simulink model "ballbeam_sim"  (Simulink 7.9)
settings: Solver=ode45  StartTime=0.0  StopTime=100  RelTol=1e-3
values from neighbouring files (symbols this model uses):
  kd_th = 2*zeta_th*wn_th/a1    [param.m]
  kd_z = -14*zeta_z*wn_z/(5*AP.g)    [param.m]
  kp_th = (AP.Fmax-Fe)/A_th    [param.m]
  kp_z = -A_th/A_z    [param.m]
undefined symbols (not defined in the file or in its folder): AP, drawBallBeam
settings Model: Creator=beard  LastModifiedBy=timmclain
settings OptimizationCC: InitFltsAndDblsToZero=on
settings DebuggingCC: FcnCallInpInsideContextMsg=Use local settings  StrictBusMsg=Warning
settings GRTTargetCC: CombineOutputUpdateFcns=off  GRTInterface=on

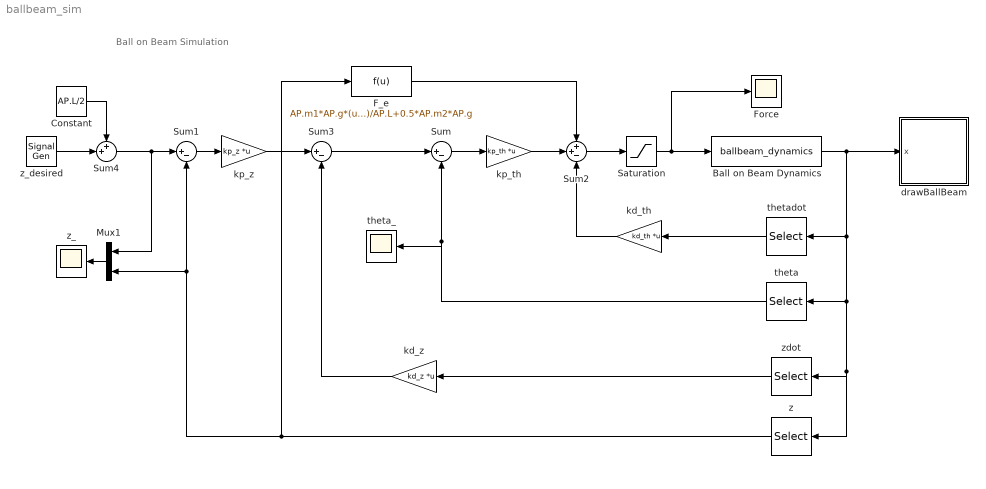
== system ballbeam_sim ==
  note: Ball on Beam Simulation
  Ball on Beam Dynamics : S-Function  FunctionName=ballbeam_dynamics  Parameters=AP  EnableBusSupport=off
  Constant : Constant  Value=AP.L/2
  F_e : Fcn  Expr=AP.m1*AP.g*(u)/AP.L+0.5*AP.m2*AP.g
  Force : Scope
      settings: TimeRange=100  YMin=6  YMax=16
  Mux1 : Mux  Inputs=2
  Saturation : Saturate  UpperLimit=AP.Fmax  LowerLimit=-AP.Fmax
  Sum : Sum  Inputs=|+-
  Sum1 : Sum  Inputs=|+-
  Sum2 : Sum  Inputs=++-
  Sum3 : Sum  Inputs=|+-
  Sum4 : Sum  Inputs=++|
  drawBallBeam : Subsystem
      mask init:
      | % drawing parameters
      | L = 0.5;
      | R = .03;
      mask Display: image(imread('tv.jpg'))
  kd_th : Gain  Gain=kd_th  Multiplication=Matrix(K*u)
  kd_z : Gain  Gain=kd_z  Multiplication=Matrix(K*u)
  kp_th : Gain  Gain=kp_th  Multiplication=Matrix(K*u)
  kp_z : Gain  Gain=kp_z  Multiplication=Matrix(K*u)
  theta : Selector  InputPortWidth=4  IndexOptions=Index vector (dialog)  Indices=[1]  OutputSizes=1
  theta_ : Scope
      settings: TimeRange=100  YMin=-0.03  YMax=0.03
  thetadot : Selector  InputPortWidth=4  IndexOptions=Index vector (dialog)  Indices=[3]  OutputSizes=1
  z : Selector  InputPortWidth=4  IndexOptions=Index vector (dialog)  Indices=[2]  OutputSizes=1
  z_ : Scope
      settings: TimeRange=100  YMin=0.05  YMax=0.45  SaveName=ScopeData2
  z_desired : SignalGenerator  WaveForm=square  Amplitude=0.15  Frequency=.02
  zdot : Selector  InputPortWidth=4  IndexOptions=Index vector (dialog)  Indices=[4]  OutputSizes=1
  wires:
  Ball on Beam Dynamics/1 -> theta/1, z/1, zdot/1, thetadot/1, drawBallBeam/1(x)
  Sum2/1 -> Saturation/1
  Sum/1 -> kp_th/1
  theta/1 -> Sum/2, theta_/1
  z/1 -> Mux1/2, Sum1/2, F_e/1
  Mux1/1 -> z_/1
  thetadot/1 -> kd_th/1
  Sum1/1 -> kp_z/1
  kp_z/1 -> Sum3/1
  zdot/1 -> kd_z/1
  kd_z/1 -> Sum3/2
  Saturation/1 -> Force/1, Ball on Beam Dynamics/1
  kd_th/1 -> Sum2/3
  kp_th/1 -> Sum2/2
  F_e/1 -> Sum2/1
  Sum3/1 -> Sum/1
  z_desired/1 -> Sum4/2
  Constant/1 -> Sum4/1
  Sum4/1 -> Sum1/1, Mux1/1

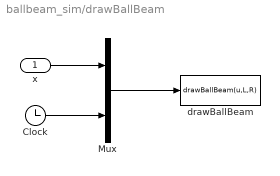
== system ballbeam_sim/drawBallBeam ==
  x : Inport
  Clock : Clock
  Mux : Mux  Inputs=2
  drawBallBeam : MATLABFcn  MATLABFcn=drawBallBeam(u,L,R)  OutputDimensions=0  SampleTime=0.1
  wires:
  Mux/1 -> drawBallBeam/1
  x/1 -> Mux/1
  Clock/1 -> Mux/2
